simulink model "Copy_of_plantaEstacionamento"  (R2023b)
settings: Solver=VariableStepAuto  StartTime=0.0  StopTime=Tf  RelTol=1e-3
values from neighbouring files (symbols this model uses):
  controlador = projetarControladorNelderMead(controlador_analitico)    [main.m]    (also in otimizacao.m = projetarControladorAnalitico(); otimizacaoCmaes.m = projetarControladorAnalitico(requisitos, planta))
  planta = obterPlantaProjeto()    [avaliarControladorAnalitico.m]    (also in calcularCusto.m = obterPlanta(); main.m = obterPlanta(); otimizacao.m; otimizacaoCmaes.m = obterPlanta())
  requisitos = obterRequisitos()    [calcularCusto.m]    (also in main.m; otimizacaoCmaes.m)
settings Model: Creator=gabri  LastModifiedBy=gubid

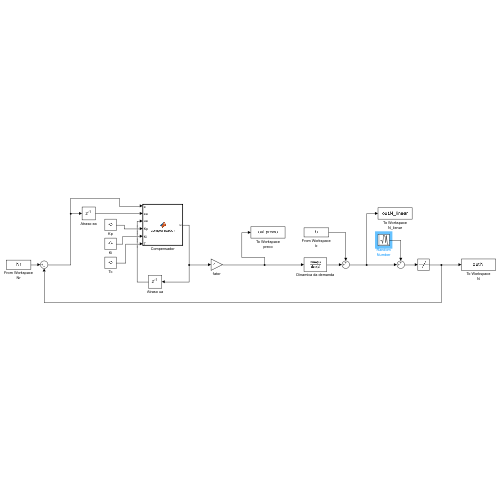
[thumbnail: Simulink's stored preview of the top-level diagram]
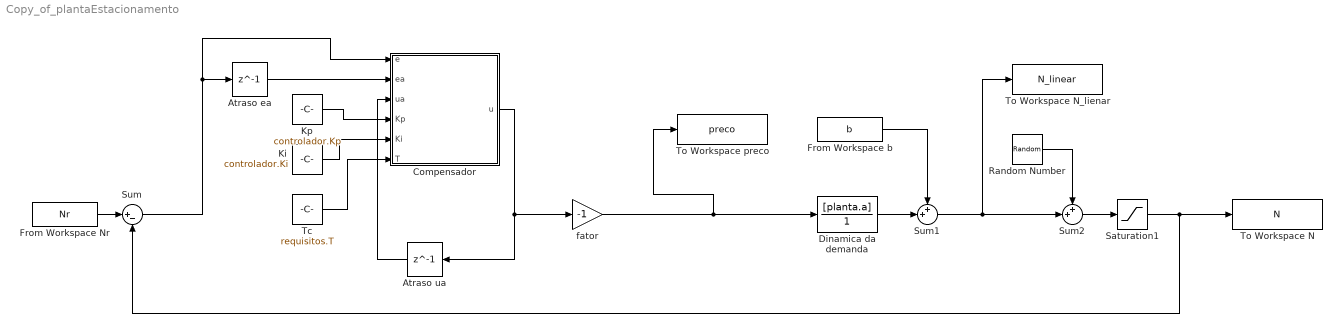
== system Copy_of_plantaEstacionamento ==
  Atraso ea : Delay  DelayLength=1  InitialCondition=0  SampleTime=requisitos.T
  Atraso ua : Delay  DelayLength=1  InitialCondition=0  SampleTime=requisitos.T
  Compensador : MATLAB Function  TreatAsAtomicUnit=on  SystemSampleTime=requisitos.T
  Dinamica da demanda : TransferFcn  Numerator=[planta.a]  Denominator=[1]
  From Workspace Nr : FromWorkspace  VariableName=Nr
  From Workspace b : FromWorkspace  VariableName=b  OutDataTypeStr=double
  Ki : Constant  Value=controlador.Ki
  Kp : Constant  Value=controlador.Kp
  Random Number : RandomNumber  Variance=planta.variancia  SampleTime=requisitos.T
  Saturation1 : Saturate  UpperLimit=1  LowerLimit=0
  Sum : Sum  Inputs=|+-
  Sum1 : Sum  Inputs=++|
  Sum2 : Sum  Inputs=++|
  Tc : Constant  Value=requisitos.T
  To Workspace N : ToWorkspace  VariableName=N  SaveFormat=Structure With Time  SampleTime=requisitos.T/100
  To Workspace N_lienar : ToWorkspace  VariableName=N_linear  SaveFormat=Structure With Time  SampleTime=requisitos.T/100
  To Workspace preco : ToWorkspace  VariableName=preco  SaveFormat=Structure With Time  SampleTime=requisitos.T/100
  fator : Gain  Gain=-1
  wires:
  Dinamica da demanda/1 -> Sum1/2
  From Workspace Nr/1 -> Sum/1
  Compensador/1(u) -> Atraso ua/1, fator/1
  From Workspace b/1 -> Sum1/1
  Sum1/1 -> To Workspace N_lienar/1, Sum2/2
  Sum2/1 -> Saturation1/1
  Random Number/1 -> Sum2/1
  Tc/1 -> Compensador/6(T)
  Sum/1 -> Compensador/1(e), Atraso ea/1
  Ki/1 -> Compensador/5(Ki)
  Atraso ua/1 -> Compensador/3(ua)
  Atraso ea/1 -> Compensador/2(ea)
  Kp/1 -> Compensador/4(Kp)
  fator/1 -> Dinamica da demanda/1, To Workspace preco/1
  Saturation1/1 -> To Workspace N/1, Sum/2

== matlab function Copy_of_plantaEstacionamento/Compensador ==
  data: e input; u output; ea input; ua input; Kp input; Ki input; T input
function u = compensador(e, ea, ua, Kp, Ki, T)
% u = compensador(e, ea, ua, Kp, Ki, T, Pmax)
% Implementa o compensador PI discreto.
% Entradas:
% e: erro atual e[k].
% ea: erro anterior e[k-1].
% ua: comando anterior u[k-1].
% Kp: ganho proporcional.
% Ki: ganho integrativo.
% T: tempo de amostragem.
% Pmax: limite de preco.
% Saidas:
% u: comando atual u[k].

u = ua + (Kp + Ki*T/2)*e + (-Kp + Ki*T/2)*ea; 

% Saturação no preço (implementação do anti-windup):
u = min(u, 0); % impedir um preço negativo (por não fazer sentido no contexto)
end
